simulink model "LQR_simulink"  (R2025b)
settings: Solver=ode45  StartTime=0.0  StopTime=5.0  RelTol=1e-3
undefined symbols (not defined in the file or in its folder): A, B, K
settings Model: Creator=alexseleznev  LastModifiedBy=alexseleznev

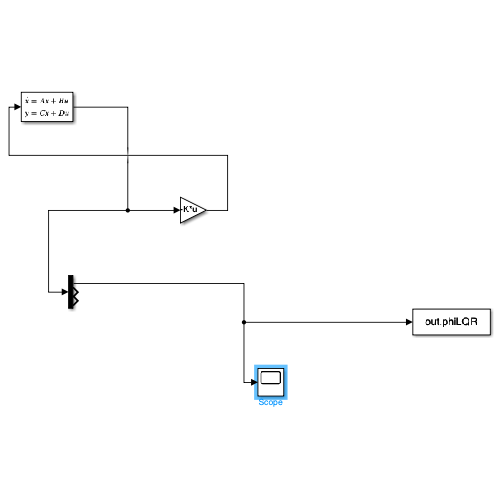
[thumbnail: Simulink's stored preview of the top-level diagram]
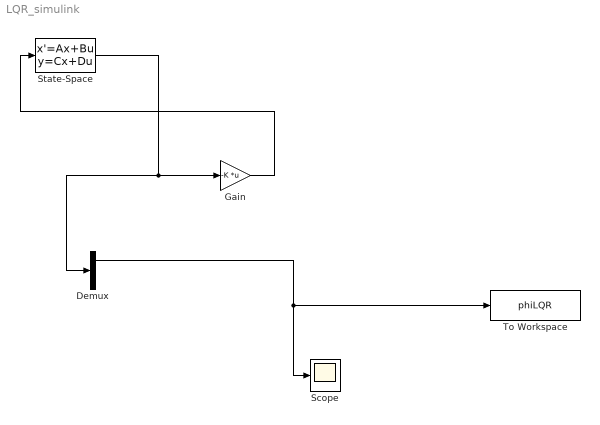
== system LQR_simulink ==
  Demux : Demux  Outputs=3
  Gain : Gain  Gain=-K  Multiplication=Matrix(K*u)
  Scope : Scope
      settings: ActiveDisplayYMinimum=-0.0062535661143483731  ActiveDisplayYMaximum=0.056269654548508338
  State-Space : StateSpace  A=A  B=B  C=eye(3)  D=zeros(3,1)  InitialCondition=[0.05; 0; 0]
  To Workspace : ToWorkspace  VariableName=phiLQR  SaveFormat=Structure With Time  SampleTime=-1
  wires:
  State-Space/1 -> Demux/1, Gain/1
  Gain/1 -> State-Space/1
  Demux/1 -> Scope/1, To Workspace/1
